simulink model "Cici_Battery_Discharge_RT"  (Simulink 8.5)
settings: Solver=ode3  StartTime=0.0  StopTime=10  FixedStep=50e-6  RelTol=1e-3
undefined symbols (not defined in the file): another_event_name, my_event_name, Q, SOC
libraries: powerlib x10, rtlab x2, artemis x1
settings Model: ARTEMISmethode_block_infos=$$__separator__$$Cici_Battery_Discharge_RT/ARTEMIS Guide$$__separator__$$  Creator=jiax  LastModifiedBy=alsetlab
settings DataIOCC: SignalLoggingSaveFormat=Dataset
settings OptimizationCC: ExpressionDepthLimit=128
settings DebuggingCC: UnderspecifiedInitializationDetection=Simplified  MergeDetectMultiDrivingBlocksExec=error  FcnCallInpInsideContextMsg=EnableAllAsError  StateNameClashWarn=none
settings GRTTargetCC: CombineOutputUpdateFcns=on  GRTInterface=off

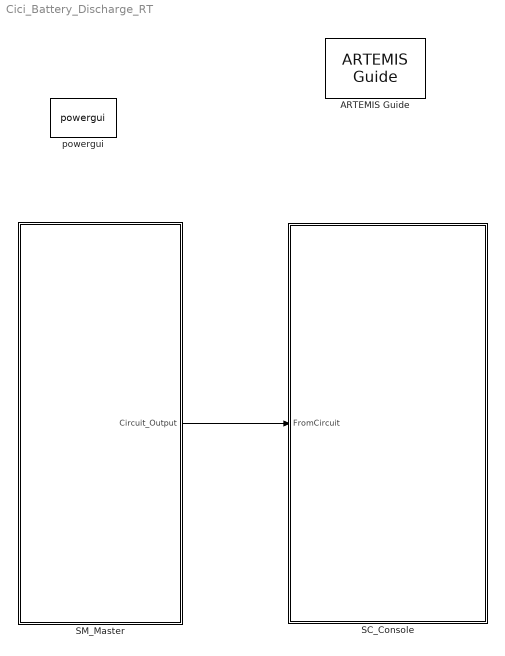
== system Cici_Battery_Discharge_RT ==
  ARTEMIS Guide : artemis/ARTEMIS/ARTEMIS Guide  Tag=FTSSmethode_opal_4hx0r99  Description=5.0_z1  lock=on  Ts=50e-6  opt=art5  dyna=off  nb_perm=4  RT_fullcomp=off  ssn=on  ssn_itvc=off  ssn_ivic=off  ssn_ext=off  ssn_solver=Art5  ssn_impulse=off  ssn_quasimpulse=off  ssn_impulse_loop=2  paraExtinctionThy=off  Thy_Impulse=on  dtc=Off  dtc_opt=normal  ao=on  simtype=off  ct_mac=off  lin_mov=off  lsp=[0.001 2]  spike_skip=Disabled  dtc_extra=1  dtc_sws=normal  dtc_pied=0.5  SPSRulesBlock=SPSRules  tre=on  ctmm=off  LF=off  dpl_type=ARTEMiS DPL  rlc_type=off  custom_type=off  para=on  ssn_ImpulseLoopBlockedStateUpdate=2  ssn_mov_iter_number=5  ssn_switch_iter_number=5  ssn_nib_type_verify=on  ssn_use_lu=on  ssn_use_ldlt=off
  SC_Console : Subsystem
  SM_Master : Subsystem
  powergui : powerlib/powergui  Priority=1  SimulationMode=Discrete  SolverType=Tustin/Backward Euler (TBE)  SampleTime=50e-6  frequency=60  SPID=off  DisableSnubberDevices=off  DisableRonSwitches=off  DisableVfSwitches=off  SwTol=0  DisplayEquations=off  Interpol=off  methode=off  Ts=100  FunctionMessages=off  echomessages=off  HookPort=off  EnableUseOfTLC=off  x0status=blocks  frequencyindice=0  Pbase=100e6  ErrMax=1e-4  Iterations=50  UnitsV=kV  UnitsW=MW  buscounter=0  RestoreLinks=warning  ResistiveCurrentMeasurement=off  Frange=[0:2:500]  Ylog=off  Xlog=on  ShowGrid=off  save=off  variable=ZData  structure=0  ZoomFFT=off  StartTime=0.0  cycles=1  DisplayStyle=1  fundamental=60  FreqAxis=off  MaxFrequency=1000  frequencyindicesteady=1  RmsSteady=1  display=off
  wires:
  SM_Master/1(Circuit_Output) -> SC_Console/1(FromCircuit)

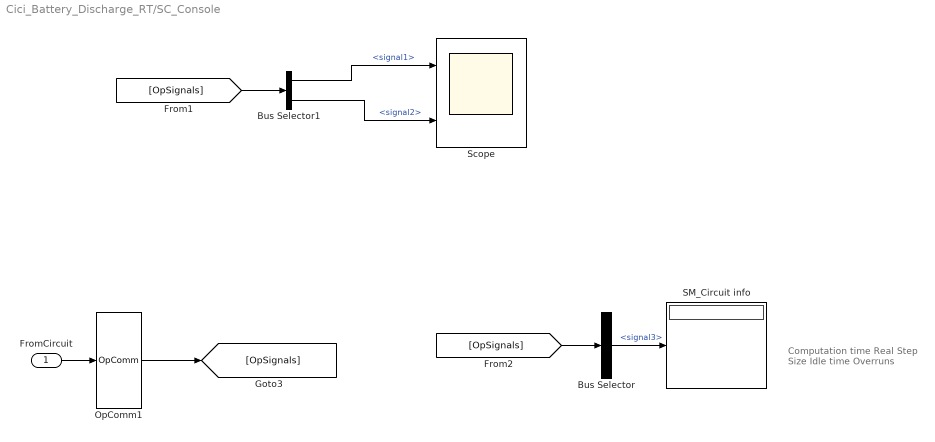
== system Cici_Battery_Discharge_RT/SC_Console ==
  note: Computation time
      | Real Step Size
      | Idle time
      | Overruns
  FromCircuit : Inport
  Bus Selector : BusSelector  OutputSignals=signal3
  Bus Selector1 : BusSelector  OutputSignals=signal1,signal2
  OpComm1 : rtlab/OpComm  nbport=1  groupe_acq=1  subsys_rate=0  st=0  Synchronization=on  Interpolation=on  Threshold=1  Missed_Data=off  Sim_Time=off  Samples=off  dynSigOut=off  from_console=0  warning_done=off  writeOpCommFile=off  Offset=off
  SM_Circuit info : Display
  Scope : Scope  NumInputPorts=2
      settings: YMin=-5~-5  YMax=5~5
  wires:
  Bus Selector/1 -> SM_Circuit info/1  "<signal3>"
  [OpSignals] -> Bus Selector/1
  OpComm1/1 -> [OpSignals]
  FromCircuit/1 -> OpComm1/1
  Bus Selector1/1 -> Scope/1  "<signal1>"
  Bus Selector1/2 -> Scope/2  "<signal2>"
  [OpSignals] -> Bus Selector1/1

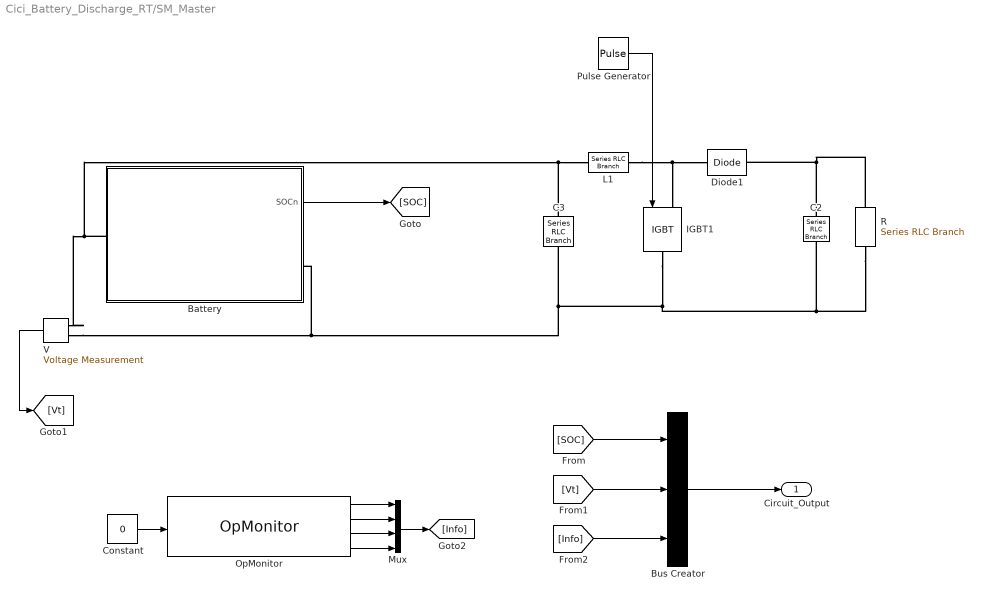
== system Cici_Battery_Discharge_RT/SM_Master ==
  Battery : Subsystem  mask{SOC0=50, capacity=10, nominal_V=3.5}
      mask prompts: SOC0 "Initial SOC"; capacity "Rated Capacity"; nominal_V "Nominla Voltage"
  Bus Creator : BusCreator  Inputs=3
  C2 : powerlib/Elements/Series RLC Branch  LConnTagsString=__new0  RConnTagsString=__new0  BranchType=C  Resistance=1.0  Inductance=1.0  SetiL0=off  InitialCurrent=0  Capacitance=100e-06  Setx0=off  InitialVoltage=0  Measurements=None
  C3 : powerlib/Elements/Series RLC Branch  LConnTagsString=__new0  RConnTagsString=__new0  BranchType=RC  Resistance=1.0  Inductance=1.0  SetiL0=off  InitialCurrent=0  Capacitance=100e-6  Setx0=off  InitialVoltage=0  Measurements=Branch voltage
  Constant : Constant  Value=0
  Diode1 : powerlib/Power Electronics/Diode  Ron=1e-4  Lon=0  Vf=0  IC=0  UseSnubber=off  Rs=inf  Cs=inf  Measurements=off
  IGBT1 : powerlib/Power Electronics/IGBT  Ron=0.001  Lon=0  Vf=0  Tf=0  Tt=0  IC=0  Rs=1e5  Cs=inf  Measurements=off
  L1 : powerlib/Elements/Series RLC Branch  LConnTagsString=__new0  RConnTagsString=__new0  BranchType=RL  Resistance=0.005  Inductance=5e-3  SetiL0=off  InitialCurrent=0  Capacitance=1e-6  Setx0=off  InitialVoltage=0  Measurements=None
  Mux : Mux
  OpMonitor : rtlab/Monitoring/OpMonitor  compute_time=on  real_step=on  idle_time=on  nb_overruns=on  user_time=off  user_name=my_event_name,another_event_name
  Pulse Generator : DiscretePulseGenerator  PulseType=Time based  Period=0.002  PulseWidth=60
  R : powerlib/Elements/Series RLC Branch  LConnTagsString=__new0  RConnTagsString=__new0  BranchType=R  Resistance=0.2  Inductance=5e-3  SetiL0=off  InitialCurrent=0  Capacitance=1e-6  Setx0=off  InitialVoltage=0  Measurements=None
  V : powerlib/Measurements/Voltage Measurement  PhasorSimulation=off  OutputType=Complex  PSBequivalent=0
  Circuit_Output : Outport
  wires:
  V/1 -> [Vt]
  Battery/1(SOCn) -> [SOC]
  Bus Creator/1 -> Circuit_Output/1
  [SOC] -> Bus Creator/1
  [Vt] -> Bus Creator/2
  Constant/1 -> OpMonitor/1
  Mux/1 -> [Info]
  OpMonitor/2 -> Mux/2
  OpMonitor/3 -> Mux/3
  OpMonitor/4 -> Mux/4
  OpMonitor/1 -> Mux/1
  [Info] -> Bus Creator/3
  Pulse Generator/1 -> IGBT1/1
  connections:
  C3/LConn1 -- Battery/LConn1 -- V/LConn1 -- L1/LConn1
  L1/RConn1 -- Diode1/LConn1 -- IGBT1/LConn1
  C2/RConn1 -- R/RConn1 -- IGBT1/RConn1 -- Battery/RConn1 -- V/LConn2 -- C3/RConn1
  R/LConn1 -- C2/LConn1 -- Diode1/RConn1

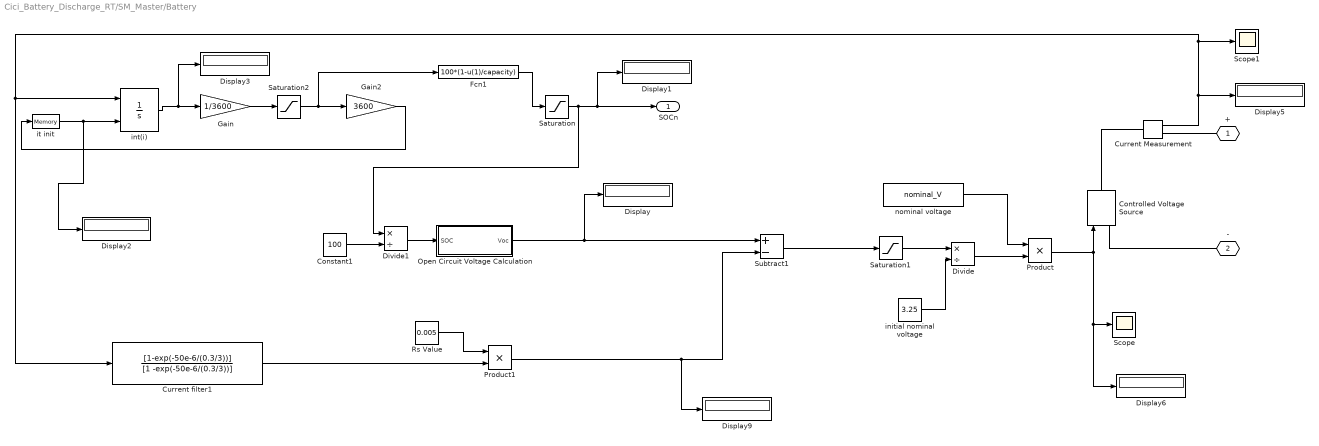
== system Cici_Battery_Discharge_RT/SM_Master/Battery ==
  Constant1 : Constant  Value=100
  Controlled Voltage Source : powerlib/Electrical Sources/Controlled Voltage Source  Initialize=on  Source_Type=AC  Amplitude=0  Phase=0  Frequency=0  Measurements=None
  Current Measurement : powerlib/Measurements/Current Measurement  PhasorSimulation=off  OutputType=Complex  PSBequivalent=0
  Current filter1 : DiscreteTransferFcn  Numerator=[1-exp(-50e-6/(0.3/3))]  Denominator=[1 -exp(-50e-6/(0.3/3))]  SampleTime=50e-6
  Display{,1..3,5..6,9} (7 alike) : Display
  Divide : Product  Inputs=*/
  Divide1 : Product  Inputs=*/
  Fcn1 : Fcn  Expr=100*(1-u(1)/capacity)
  Gain : Gain  Gain=1/3600
  Gain2 : Gain  Gain=3600
  Open Circuit Voltage Calculation : Subsystem
  Product : Product
  Product1 : Product
  Rs Value : Constant  Value=0.005
  Saturation : Saturate  UpperLimit=100  LowerLimit=0
  Saturation1 : Saturate  UpperLimit=10  LowerLimit=0
  Saturation2 : Saturate  UpperLimit=capacity*0.9999  LowerLimit=0
  Scope : Scope
      settings: YMin=6.89401  YMax=6.89404  SaveName=Cici_Battery_Voltage_Charge
  Scope1 : Scope
      settings: YMin=-91.795  YMax=-91.77
  Subtract1 : Sum  Inputs=+-
  initial nominal voltage : Constant  Value=3.25
  int(i) : Integrator  InitialConditionSource=external  InitialCondition=(1-SOC/100)*Q*3600  LimitOutput=on  UpperSaturationLimit=capacity*3600
  it init : Memory  X0=(1-SOC0/100)*capacity*3600
  nominal voltage : Constant  Value=nominal_V
  + : PMIOPort  Tag=PMCPort  Port=1  Side=Left
  - : PMIOPort  Tag=PMCPort  Port=2  Side=Right
  SOCn : Outport
  wires:
  Saturation/1 -> Display1/1, SOCn/1, Divide1/1
  Open Circuit Voltage Calculation/1(Voc) -> Display/1, Subtract1/1
  Current Measurement/1 -> Scope1/1, Current filter1/1, int(i)/1, Display5/1
  Product1/1 -> Display9/1, Subtract1/2
  Divide/1 -> Product/2
  Product/1 -> Controlled Voltage Source/1, Display6/1, Scope/1
  initial nominal voltage/1 -> Divide/2
  Saturation1/1 -> Divide/1
  Subtract1/1 -> Saturation1/1
  Rs Value/1 -> Product1/1
  int(i)/1 -> Display3/1, Gain/1
  Gain/1 -> Saturation2/1
  Saturation2/1 -> Fcn1/1, Gain2/1
  Gain2/1 -> it init/1
  Fcn1/1 -> Saturation/1
  nominal voltage/1 -> Product/1
  Divide1/1 -> Open Circuit Voltage Calculation/1(SOC)
  Constant1/1 -> Divide1/2
  it init/1 -> Display2/1, int(i)/2
  Current filter1/1 -> Product1/2
  connections:
  Current Measurement/RConn1 -- +/RConn1
  Controlled Voltage Source/LConn1 -- -/RConn1
  Current Measurement/LConn1 -- Controlled Voltage Source/RConn1

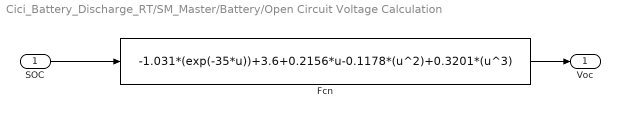
== system Cici_Battery_Discharge_RT/SM_Master/Battery/Open Circuit Voltage Calculation ==
  SOC : Inport
  Fcn : Fcn  Expr=-1.031*(exp(-35*u))+3.6+0.2156*u-0.1178*(u^2)+0.3201*(u^3)
  Voc : Outport
  wires:
  SOC/1 -> Fcn/1
  Fcn/1 -> Voc/1
